simulink model "DCsimq3"  (R2014a)
settings: Solver=ode45  StartTime=0.0  StopTime=2  RelTol=1e-3
values from neighbouring files (symbols this model uses):
  Beff = Bmk + Kbk*Kmk/Rk    (= 1.51875e-06)    [scriptQ3.m]
  Jeff = Jmk +dkk/(r)^2    (= 3.01e-06)    [scriptQ3.m]
  K = 1    [scriptQ3.m]
  KD1 = (2*zeta*w*Jeff-Beff)/K*set1(2)    [scriptQ3.m]
  KD2 = KD1    [scriptQ3.m]
  KD3 = (2*zeta*w*Jeff-Beff)/K*set2(2)    [scriptQ3.m]
  KD4 = KD3    [scriptQ3.m]
  KD5 = (2*zeta*w*Jeff-Beff)/K*set3(2)    [scriptQ3.m]
  KD6 = KD5    [scriptQ3.m]
  KI1 = (Beff+K*KD1)*KP1/Jeff*set1(3)    [scriptQ3.m]
  KI2 = KI1    [scriptQ3.m]
  KI3 = (Beff+K*KD3)*KP3/Jeff*set2(3)    [scriptQ3.m]
  KI4 = KI3    [scriptQ3.m]
  KI5 = (Beff+K*KD5)*KP5/Jeff*set3(3)    [scriptQ3.m]
  KI6 = KI5    [scriptQ3.m]
  KP1 = w^2*Jeff/K*set1(1)    [scriptQ3.m]
  KP2 = KP1    [scriptQ3.m]
  KP3 = w^2*Jeff/K*set2(1)    [scriptQ3.m]
  KP4 = KP3    [scriptQ3.m]
  KP5 = w^2*Jeff/K*set3(1)    [scriptQ3.m]
  KP6 = KP5    [scriptQ3.m]
settings Model: Creator=Retta  LastModifiedBy=Retta

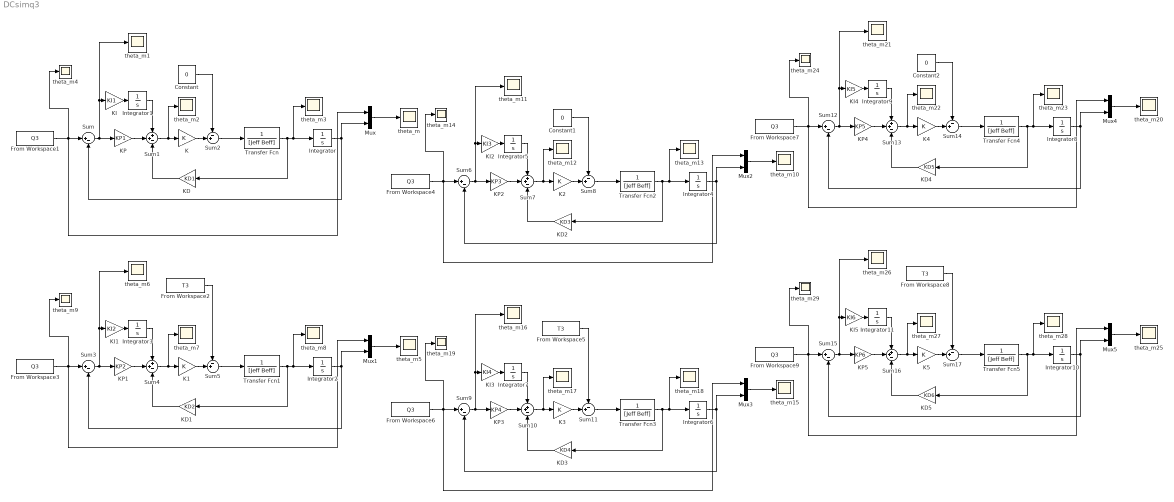
== system DCsimq3 ==
  Constant : Constant  Value=0
  Constant1 : Constant  Value=0
  Constant2 : Constant  Value=0
  From Workspace{1,3..4,6..7,9} (6 alike) : FromWorkspace  VariableName=Q3  SampleTime=0
  From Workspace2 : FromWorkspace  VariableName=T3  SampleTime=0
  From Workspace5 : FromWorkspace  VariableName=T3  SampleTime=0
  From Workspace8 : FromWorkspace  VariableName=T3  SampleTime=0
  Integrator{,1..11} (12 alike) : Integrator
  K{,1..5} (6 alike) : Gain  Gain=K
  KD : Gain  Gain=KD1
  KD1 : Gain  Gain=KD2
  KD2 : Gain  Gain=KD3
  KD3 : Gain  Gain=KD4
  KD4 : Gain  Gain=KD5
  KD5 : Gain  Gain=KD6
  KI : Gain  Gain=KI1
  KI1 : Gain  Gain=KI2
  KI2 : Gain  Gain=KI3
  KI3 : Gain  Gain=KI4
  KI4 : Gain  Gain=KI5
  KI5 : Gain  Gain=KI6
  KP : Gain  Gain=KP1
  KP1 : Gain  Gain=KP2
  KP2 : Gain  Gain=KP3
  KP3 : Gain  Gain=KP4
  KP4 : Gain  Gain=KP5
  KP5 : Gain  Gain=KP6
  Mux{,1..5} (6 alike) : Mux  Inputs=2
  Sum{,3,6,9,12,15} (6 alike) : Sum  Inputs=|+-
  Sum{1,4,7,10,13,16} (6 alike) : Sum  Inputs=++-
  Sum{2,5,8,11,14,17} (6 alike) : Sum  Inputs=-+|
  Transfer Fcn{,1..5} (6 alike) : TransferFcn  Denominator=[Jeff Beff]
  theta_m{,1..29} (30 alike) : Scope
      theta_m settings: TimeRange=10  YMin=0  YMax=0.5  SaveName=ver1
      theta_m10 settings: TimeRange=10  YMin=0  YMax=0.5  SaveName=ver3
      theta_m11 settings: SaveName=ScopeData8
      theta_m12 settings: SaveName=ScopeData9
      theta_m13 settings: SaveName=ScopeData10
      theta_m14 settings: SaveName=ScopeData11
      theta_m15 settings: TimeRange=10  YMin=0  YMax=0.5  SaveName=ver4
      theta_m16 settings: SaveName=ScopeData12
      theta_m17 settings: SaveName=ScopeData13
      theta_m18 settings: SaveName=ScopeData14
      theta_m19 settings: SaveName=ScopeData15
      theta_m2 settings: SaveName=ScopeData2
      theta_m20 settings: TimeRange=10  YMin=0  YMax=0.5  SaveName=ver5
      theta_m21 settings: SaveName=ScopeData16
      theta_m22 settings: SaveName=ScopeData17
      theta_m23 settings: SaveName=ScopeData18
      theta_m24 settings: SaveName=ScopeData19
      theta_m25 settings: TimeRange=10  YMin=0  YMax=0.5  SaveName=ver6
      theta_m26 settings: SaveName=ScopeData20
      theta_m27 settings: SaveName=ScopeData21
      theta_m28 settings: SaveName=ScopeData22
      theta_m29 settings: SaveName=ScopeData23
      theta_m3 settings: SaveName=ScopeData3
      theta_m4 settings: SaveName=ScopeData4
      theta_m5 settings: TimeRange=10  YMin=0  YMax=0.5  SaveName=ver2
      theta_m7 settings: SaveName=ScopeData5
      theta_m8 settings: SaveName=ScopeData6
      theta_m9 settings: SaveName=ScopeData7
  wires:
  From Workspace1/1 -> theta_m4/1, Mux/1, Sum/1
  Sum/1 -> theta_m1/1, KI/1, KP/1
  Sum1/1 -> theta_m2/1, K/1
  K/1 -> Sum2/2
  Sum2/1 -> Transfer Fcn/1
  Transfer Fcn/1 -> theta_m3/1, Integrator/1, KD/1
  Integrator/1 -> Mux/2, Sum/2
  KD/1 -> Sum1/3
  KP/1 -> Sum1/2
  KI/1 -> Integrator1/1
  Integrator1/1 -> Sum1/1
  Mux/1 -> theta_m/1
  Constant/1 -> Sum2/1
  From Workspace3/1 -> theta_m9/1, Mux1/1, Sum3/1
  Sum3/1 -> theta_m6/1, KI1/1, KP1/1
  Sum4/1 -> theta_m7/1, K1/1
  K1/1 -> Sum5/2
  Sum5/1 -> Transfer Fcn1/1
  Transfer Fcn1/1 -> theta_m8/1, Integrator2/1, KD1/1
  Integrator2/1 -> Mux1/2, Sum3/2
  KD1/1 -> Sum4/3
  KP1/1 -> Sum4/2
  KI1/1 -> Integrator3/1
  Integrator3/1 -> Sum4/1
  Mux1/1 -> theta_m5/1
  From Workspace2/1 -> Sum5/1
  From Workspace4/1 -> theta_m14/1, Mux2/1, Sum6/1
  Sum6/1 -> theta_m11/1, KI2/1, KP2/1
  Sum7/1 -> theta_m12/1, K2/1
  K2/1 -> Sum8/2
  Sum8/1 -> Transfer Fcn2/1
  Transfer Fcn2/1 -> theta_m13/1, Integrator4/1, KD2/1
  Integrator4/1 -> Mux2/2, Sum6/2
  KD2/1 -> Sum7/3
  KP2/1 -> Sum7/2
  KI2/1 -> Integrator5/1
  Integrator5/1 -> Sum7/1
  Mux2/1 -> theta_m10/1
  Constant1/1 -> Sum8/1
  From Workspace6/1 -> theta_m19/1, Mux3/1, Sum9/1
  Sum9/1 -> theta_m16/1, KI3/1, KP3/1
  Sum10/1 -> theta_m17/1, K3/1
  K3/1 -> Sum11/2
  Sum11/1 -> Transfer Fcn3/1
  Transfer Fcn3/1 -> theta_m18/1, Integrator6/1, KD3/1
  Integrator6/1 -> Mux3/2, Sum9/2
  KD3/1 -> Sum10/3
  KP3/1 -> Sum10/2
  KI3/1 -> Integrator7/1
  Integrator7/1 -> Sum10/1
  Mux3/1 -> theta_m15/1
  From Workspace5/1 -> Sum11/1
  From Workspace7/1 -> theta_m24/1, Mux4/1, Sum12/1
  Sum12/1 -> theta_m21/1, KI4/1, KP4/1
  Sum13/1 -> theta_m22/1, K4/1
  K4/1 -> Sum14/2
  Sum14/1 -> Transfer Fcn4/1
  Transfer Fcn4/1 -> theta_m23/1, Integrator8/1, KD4/1
  Integrator8/1 -> Mux4/2, Sum12/2
  KD4/1 -> Sum13/3
  KP4/1 -> Sum13/2
  KI4/1 -> Integrator9/1
  Integrator9/1 -> Sum13/1
  Mux4/1 -> theta_m20/1
  Constant2/1 -> Sum14/1
  From Workspace9/1 -> theta_m29/1, Mux5/1, Sum15/1
  Sum15/1 -> theta_m26/1, KI5/1, KP5/1
  Sum16/1 -> theta_m27/1, K5/1
  K5/1 -> Sum17/2
  Sum17/1 -> Transfer Fcn5/1
  Transfer Fcn5/1 -> theta_m28/1, Integrator10/1, KD5/1
  Integrator10/1 -> Mux5/2, Sum15/2
  KD5/1 -> Sum16/3
  KP5/1 -> Sum16/2
  KI5/1 -> Integrator11/1
  Integrator11/1 -> Sum16/1
  Mux5/1 -> theta_m25/1
  From Workspace8/1 -> Sum17/1
